simulink model "abc"  (R2020b)
settings: Solver=VariableStepAuto  StartTime=0.0  StopTime=10.0  RelTol=1e-3
libraries: cm_custom x1
settings Model: Creator=Ray  LastModifiedBy=Ray

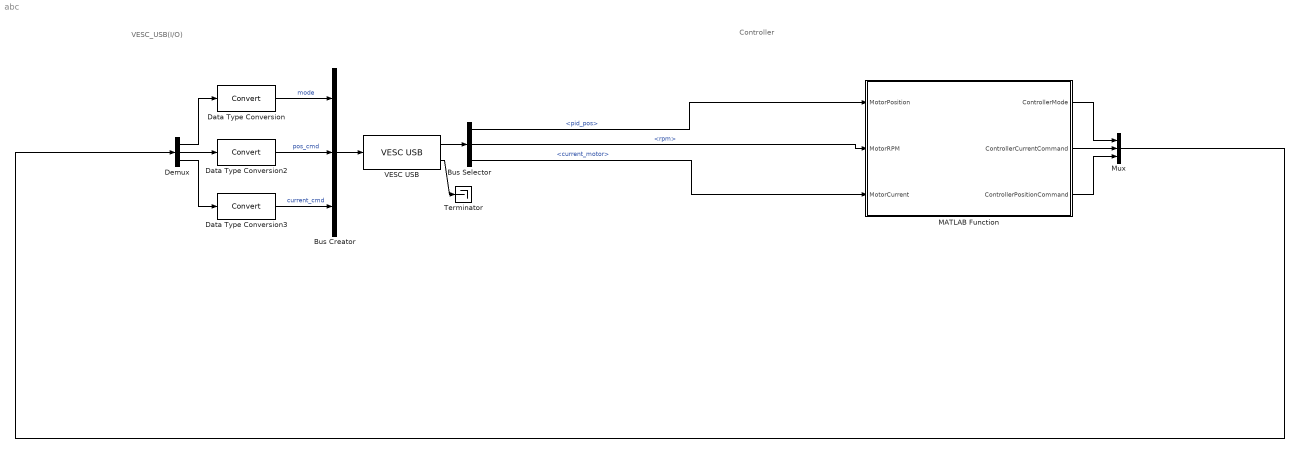
== system abc ==
  note: Controller
  note: VESC_USB(I/O)
  Bus Creator : BusCreator  Inputs=3
  Bus Selector : BusSelector  OutputSignals=pid_pos,rpm,current_motor
  Data Type Conversion : DataTypeConversion
  Data Type Conversion2 : DataTypeConversion
  Data Type Conversion3 : DataTypeConversion
  Demux : Demux  Outputs=3
  MATLAB Function : MATLAB Function  TreatAsAtomicUnit=on
  Mux : Mux  Inputs=3
  Terminator : Terminator
  VESC USB : cm_custom/VESC USB  PAR_VESC_DEV='/dev/VESC_SFB_1'  POS_KP=0.001  POS_KI=0  POS_KD=0.001  POS_KD_FIL=0.2  POS_DIV=1  CURR_MAX=20  CURR_MIN=-20  CURR_IN_MAX=20  CURR_IN_MIN=-20  CURR_ABS_MAX=20  PAR_SMPLT=0.05
      link override S-Function Builder5: Parameters=uint8(PAR_VESC_DEV)  FunctionName=sf_vesc_usb
  wires:
  Bus Creator/1 -> VESC USB/1
  VESC USB/2 -> Terminator/1
  VESC USB/1 -> Bus Selector/1
  Data Type Conversion/1 -> Bus Creator/1  "mode"
  Data Type Conversion3/1 -> Bus Creator/3  "current_cmd"
  Data Type Conversion2/1 -> Bus Creator/2  "pos_cmd"
  Bus Selector/2 -> MATLAB Function/2(MotorRPM)  "<rpm>"
  Bus Selector/1 -> MATLAB Function/1(MotorPosition)  "<pid_pos>"
  Bus Selector/3 -> MATLAB Function/3(MotorCurrent)  "<current_motor>"
  MATLAB Function/1(ControllerMode) -> Mux/1
  MATLAB Function/2(ControllerCurrentCommand) -> Mux/2
  MATLAB Function/3(ControllerPositionCommand) -> Mux/3
  Mux/1 -> Demux/1
  Demux/2 -> Data Type Conversion2/1
  Demux/1 -> Data Type Conversion/1
  Demux/3 -> Data Type Conversion3/1

== matlab function abc/MATLAB Function ==
  data: MotorPosition input; ControllerMode output; ControllerCurrentCommand output; ControllerPositionCommand output; MotorRPM input; MotorCurrent input
function [ControllerMode,ControllerCurrentCommand,ControllerPositionCommand]= fcn(MotorPosition,MotorRPM,MotorCurrent)

y = u;
